simulink library "stimulation_visual_lib"  (Simulink 4.00)
settings Model: LastModifiedBy=bsaunder

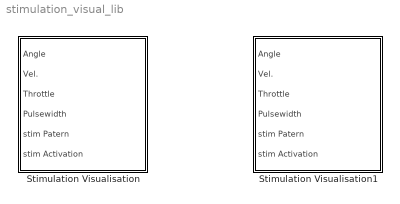
== system stimulation_visual_lib ==
  Stimulation Visualisation : Subsystem  mask{show=on, Ts=0.05}
      mask prompts: show "Show the animation window"; Ts "Sample time"
      mask help: This block provides a visualisation of the cycling action, stimulation pattern and stimulation activation as well as providing read outs of the angle, angular velocity, throttle value and stimulation value.
      settings: RTWFcnNameOpts=Auto  RTWFileNameOpts=Auto
      mask Display:
      | port_label('input', 1, 'Angle');
      | port_label('input', 2, 'Vel.');
      | port_label('input', 3, 'Throttle');
      | port_label('input', 4, 'Pulsewidth');
      | port_label('input', 5, 'Stimulation Pattern');
      | port_label('input', 6, 'Stimulation Activation');
      | 
      | plot((0.4.*sin([0:pi/180:2*pi]))+0.5, (0.4.*cos([0:pi/180:2*pi]))+0.5);
      | 
      | plot((0.3.*sin([10*(pi/180):pi/180:110*(pi/180)]))+0.5, (0.3.*cos([10*(pi/180):pi/180:110*(pi/180)]))+0.5);
      | plot((0.3.*sin([190*(pi/180):pi/180:290*(pi/180)]))+0.5, (0.3.*cos([190*(pi/180):pi/180:290*(pi/180)]))+0.5);
      | 
      | plot((0.2.*sin([60*(pi/180):pi/180:160*(pi/180)]))+0.5, (0.2.*cos([60*(pi/180):pi/180:160*(pi/180)]))+0.5);
      | plot((0.2.*sin([240*(pi/180):pi/180:340*(pi/180)]))+0.5, (0.2.*cos([240*(pi/180):pi/180:340*(pi/180)]))+0.5);
      | 
      | plot((0.1.*sin([-30*(pi/180):pi/180:30*(pi/180)]))+0.5, (0.1.*cos([-30*(pi/180):pi/180:30*(pi/180)]))+0.5);
      | plot((0.1.*sin([150*(pi/180):pi/180:210*(pi/180)]))+0.5, (0.1.*cos([150*(pi/180):pi/180:210*(pi/180)]))+0.5);
  Stimulation Visualisation1 : Subsystem  mask{show=on, Ts=0.05}
      mask prompts: show "Show the animation window"; Ts "Sample time"
      mask help: This block provides a visualisation of the cycling action, stimulation pattern and stimulation activation as well as providing read outs of the angle, angular velocity, throttle value and stimulation value.
      settings: RTWFcnNameOpts=Auto  RTWFileNameOpts=Auto
      mask Display:
      | port_label('input', 1, 'Angle');
      | port_label('input', 2, 'Vel.');
      | port_label('input', 3, 'Throttle');
      | port_label('input', 4, 'Pulsewidth');
      | port_label('input', 5, 'Stimulation Pattern');
      | port_label('input', 6, 'Stimulation Activation');
      | 
      | plot((0.4.*sin([0:pi/180:2*pi]))+0.5, (0.4.*cos([0:pi/180:2*pi]))+0.5);
      | 
      | plot((0.3.*sin([10*(pi/180):pi/180:110*(pi/180)]))+0.5, (0.3.*cos([10*(pi/180):pi/180:110*(pi/180)]))+0.5);
      | plot((0.3.*sin([190*(pi/180):pi/180:290*(pi/180)]))+0.5, (0.3.*cos([190*(pi/180):pi/180:290*(pi/180)]))+0.5);
      | 
      | plot((0.2.*sin([60*(pi/180):pi/180:160*(pi/180)]))+0.5, (0.2.*cos([60*(pi/180):pi/180:160*(pi/180)]))+0.5);
      | plot((0.2.*sin([240*(pi/180):pi/180:340*(pi/180)]))+0.5, (0.2.*cos([240*(pi/180):pi/180:340*(pi/180)]))+0.5);
      | 
      | plot((0.1.*sin([-30*(pi/180):pi/180:30*(pi/180)]))+0.5, (0.1.*cos([-30*(pi/180):pi/180:30*(pi/180)]))+0.5);
      | plot((0.1.*sin([150*(pi/180):pi/180:210*(pi/180)]))+0.5, (0.1.*cos([150*(pi/180):pi/180:210*(pi/180)]))+0.5);
      | 
      | text(0.5, 0.5, 'Movie', 'HorizontalAlignment', 'center')

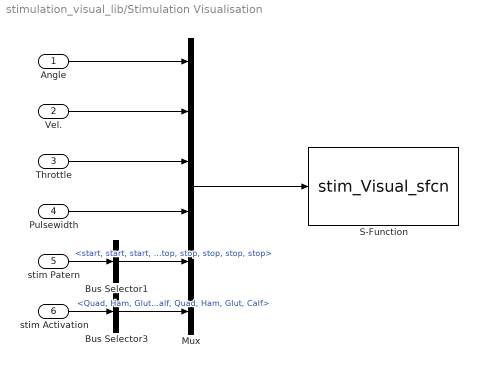
== system stimulation_visual_lib/Stimulation Visualisation ==
  Angle : Inport  Port=1  LatchInput=off
  Vel. : Inport  Port=2  LatchInput=off
  Throttle : Inport  Port=3  LatchInput=off
  Pulsewidth : Inport  Port=4  LatchInput=off
  stim Patern : Inport  Port=5  LatchInput=off
  stim Activation : Inport  Port=6  LatchInput=off
  Bus Selector1 : BusSelector  OutputSignals=R.Quad.start,R.Ham.start,R.Glut.start,R.Calf.start,L.Quad.start,L.Ham.start,L.Glut.start,L.Calf.start,R.Quad.stop,R.Ham.stop,R.Glut.stop,R.Calf.stop,L.Quad.stop,L.Ham.stop,L.Glut.stop,L.Calf.stop  MuxedOutput=on
  Bus Selector3 : BusSelector  OutputSignals=R.Quad,R.Ham,R.Glut,R.Calf,L.Quad,L.Ham,L.Glut,L.Calf  MuxedOutput=on
  Mux : Mux  Inputs=6
  S-Function : S-Function  FunctionName=stim_Visual_sfcn  Parameters=Ts, show  PortCounts=[]  SFunctionModules=''
  wires:
  Mux/1 -> S-Function/1
  Bus Selector3/1 -> Mux/6  "<Quad, Ham, Glut, Calf, Quad, Ham, Glut, Calf>"
  Bus Selector1/1 -> Mux/5  "<start, start, start, start, start, start, start, start, stop, stop, stop, stop, stop, stop, stop, stop>"
  Pulsewidth/1 -> Mux/4
  Throttle/1 -> Mux/3
  Vel./1 -> Mux/2
  Angle/1 -> Mux/1
  stim Activation/1 -> Bus Selector3/1
  stim Patern/1 -> Bus Selector1/1

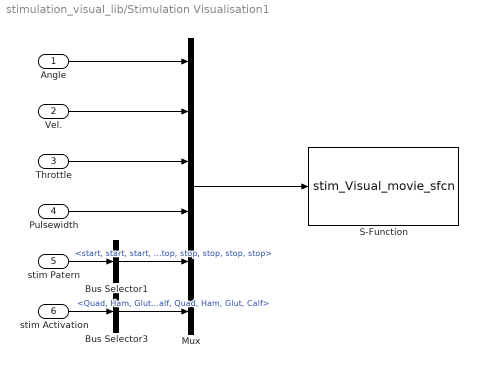
== system stimulation_visual_lib/Stimulation Visualisation1 ==
  Angle : Inport  Port=1  LatchInput=off
  Vel. : Inport  Port=2  LatchInput=off
  Throttle : Inport  Port=3  LatchInput=off
  Pulsewidth : Inport  Port=4  LatchInput=off
  stim Patern : Inport  Port=5  LatchInput=off
  stim Activation : Inport  Port=6  LatchInput=off
  Bus Selector1 : BusSelector  OutputSignals=R.Quad.start,R.Ham.start,R.Glut.start,R.Calf.start,L.Quad.start,L.Ham.start,L.Glut.start,L.Calf.start,R.Quad.stop,R.Ham.stop,R.Glut.stop,R.Calf.stop,L.Quad.stop,L.Ham.stop,L.Glut.stop,L.Calf.stop  MuxedOutput=on
  Bus Selector3 : BusSelector  OutputSignals=R.Quad,R.Ham,R.Glut,R.Calf,L.Quad,L.Ham,L.Glut,L.Calf  MuxedOutput=on
  Mux : Mux  Inputs=6
  S-Function : S-Function  FunctionName=stim_Visual_movie_sfcn  Parameters=Ts, show  PortCounts=[]  SFunctionModules=''
  wires:
  stim Patern/1 -> Bus Selector1/1
  stim Activation/1 -> Bus Selector3/1
  Angle/1 -> Mux/1
  Vel./1 -> Mux/2
  Throttle/1 -> Mux/3
  Pulsewidth/1 -> Mux/4
  Bus Selector1/1 -> Mux/5  "<start, start, start, start, start, start, start, start, stop, stop, stop, stop, stop, stop, stop, stop>"
  Bus Selector3/1 -> Mux/6  "<Quad, Ham, Glut, Calf, Quad, Ham, Glut, Calf>"
  Mux/1 -> S-Function/1
